simulink model "s9_3"  (R2024a)
settings: Solver=ode23  StartTime=0.0  StopTime=t_d  MaxStep=Tc  RelTol=1e-8  AbsTol=1e-8
model workspace: external: MAT-File C:\Users\tatwi\Documents\GitHub\robot_sim\Impedance_Control\test.mat (data not in the file)
values from neighbouring files (symbols this model uses):
  a = str2num(a_Field.Value)    [ImpedanceButton_Callback.m]    (also in i9_a_Backup.m = [1;1]; impedanceControl_ws.mat = [2 1]; param.m = [1;1]; test.mat = [1 1])
  F_v = K_r*diag([0.01 0.01])*K_r    [ImpedanceButton_Callback.m]    (also in i9_3.m; i9_a_Backup.m; impedanceControl_ws.mat = [100  0; 0  100]; test.mat = [100  0; 0  100])
  g = str2num(g_Field.Value)    [ImpedanceButton_Callback.m]    (also in i9_3.m = 9.81; i9_a_Backup.m = 9.81; impedanceControl_ws.mat = 9.81; test.mat = 9.81)
  iM_d = inv(M_d)    [ImpedanceButton_Callback.m]    (also in i9_3.m; i9_a_Backup.m; impedanceControl_ws.mat = [0.01  0; 0  0.01]; test.mat = [0.01  0; 0  0.01])
  K = R_c*[0 0;0 5e3]*R_c'    [ImpedanceButton_Callback.m]    (also in i9_3.m; i9_a_Backup.m; impedanceControl_ws.mat = [2500  -2500; -2500  2500]; test.mat = [2500  -2500; -2500  2500])
  K_d = Kd*diag([1 1])    [ImpedanceButton_Callback.m]    (also in i9_3.m = 1600*diag([1 1]); i9_a_Backup.m = 1600*diag([1 1]); impedanceControl_ws.mat = [1600  0; 0  1600]; test.mat = [1600  0; 0  1600])
  K_p = Kp*diag([1 1])    [ImpedanceButton_Callback.m]    (also in i9_3.m = 5000*diag([1 1]); i9_a_Backup.m = 5000*diag([1 1]); impedanceControl_ws.mat = [5000  0; 0  5000]; test.mat = [5000  0; 0  5000])
  o_r = [1;0]    [ImpedanceButton_Callback.m]    (also in i9_3.m; i9_a_Backup.m; impedanceControl_ws.mat = [1 0]; test.mat = [1 0])
  pi_l = pi_m    [ImpedanceButton_Callback.m]    (also in i9_3.m; i9_a_Backup.m; impedanceControl_ws.mat = [135 72.51 25 -2.5 0.01]; test.mat = [80 97.51 25 -2.5 0.01])
  pi_m = [135 72.51 25 -2.5 0.01]    [impedanceControl_ws.mat]    (also in test.mat = [80 97.51 25 -2.5 0.01])
  q_i = inv_k2u(a,p_i)    [ImpedanceButton_Callback.m]    (also in i9_3.m; i9_a_Backup.m; impedanceControl_ws.mat = [0.340969724421 -2.74996579108]; test.mat = [0.963425266026 -1.92685053205])
  Tc = str2num(tc_Field.Value)    [ImpedanceButton_Callback.m]    (also in i9_3.m = 0.001; i9_a_Backup.m = 0.001; impedanceControl_ws.mat = 0.001; test.mat = 0.001)
  Ts = Tc    [ImpedanceButton_Callback.m]    (also in i9_3.m = 0.001; i9_a_Backup.m = 0.001; impedanceControl_ws.mat = 0.001; test.mat = 0.001)
undefined symbols (not defined in the file or in its folder): iner, iner_l
settings Model: Creator=luigivillani  LastModifiedBy=tatwi
settings SolverCC: AutoScaleAbsTol=off  AlgebraicLoopSolver=TrustRegion
settings DataIOCC: SaveFormat=Array  SignalLoggingSaveFormat=ModelDataLogs  SaveOutput=off  SaveTime=off  ReturnWorkspaceOutputs=off
settings OptimizationCC: BlockReduction=off  BooleanDataType=off  ExpressionDepthLimit=2147483647  InitFltsAndDblsToZero=on  LifeSpan=inf
settings DebuggingCC: SaveWithParameterizedLinksMsg=none  UnderspecifiedInitializationDetection=Classic  MergeDetectMultiDrivingBlocksExec=none  SignalResolutionControl=TryResolveAllWithWarning  MultiTaskDSMMsg=warning  MultiTaskCondExecSysMsg=none  FcnCallInpInsideContextMsg=warning  UnconnectedInputMsg=warning  UnconnectedOutputMsg=warning  UnconnectedLineMsg=warning  StateNameClashWarn=warning  SFUnexpectedBacktrackingDiag=warning  SFNoUnconditionalDefaultTransitionDiag=warning  SFExecutionAtInitializationDiag=none  ArithmeticOperatorsInVariantConditions=warning
settings HardwareCC: ProdBitPerPointer=32  ProdBitPerSizeT=32  ProdBitPerPtrDiffT=32  ProdLargestAtomicFloat=None  ProdIntDivRoundTo=Undefined  ProdEndianess=Unspecified  ProdWordSize=32  ProdHWDeviceType=32-bit Generic  TargetUnknown=on
settings ModelReferenceCC: PropagateSignalLabelsOutOfModel=off
settings RTWCC: GPUComputeCapability=3.5
settings CodeAppCC: StateflowObjectComments=on
settings GRTTargetCC: TargetFcnLib=ansi_tfl_tmw.mat  TargetLangStandard=C89/C90 (ANSI)  CombineOutputUpdateFcns=off  GRTInterface=on
settings ConfigComp: CovMetricSettings=dw  CovSaveCumulativeToWorkspaceVar=on  CovSaveSingleToWorkspaceVar=on

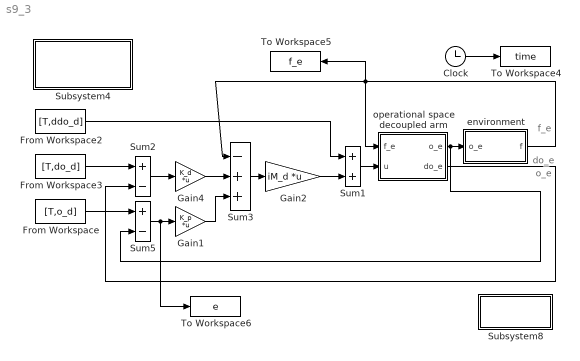
== system s9_3 ==
  note: o_e
  note: do_e
  note: f_e
  Clock : Clock
  From Workspace : FromWorkspace  VariableName=[T,o_d]  SampleTime=Tc  ZeroCross=off
  From Workspace2 : FromWorkspace  VariableName=[T,ddo_d]  SampleTime=Tc  ZeroCross=off
  From Workspace3 : FromWorkspace  VariableName=[T,do_d]  SampleTime=Tc  ZeroCross=off
  Gain1 : Gain  Gain=K_p  Multiplication=Matrix(K*u)  SampleTime=Tc
      mask Display: disp('K_p')
  Gain2 : Gain  Gain=iM_d  Multiplication=Matrix(K*u)  SampleTime=Tc
      mask Display: disp('inv(M_d)')
  Gain4 : Gain  Gain=K_d  Multiplication=Matrix(K*u)  SampleTime=Tc
      mask Display: disp('K_d')
  Subsystem4 : Subsystem
      settings: OpenFcn=clear all;i9_3;
      mask Display: disp('variables\ninitialization')
  Subsystem8 : Subsystem
      settings: OpenFcn=p9_3;
      mask Display: disp('plot')
  Sum1 : Sum  InputSameDT=on  SaturateOnIntegerOverflow=on  OutDataTypeStr=Inherit: Same as first input
  Sum2 : Sum  Inputs=+-  InputSameDT=on  SaturateOnIntegerOverflow=on  SampleTime=Tc  OutDataTypeStr=Inherit: Same as first input
  Sum3 : Sum  Inputs=-++  InputSameDT=on  SaturateOnIntegerOverflow=on  SampleTime=Tc  OutDataTypeStr=Inherit: Same as first input
  Sum5 : Sum  Inputs=+-  InputSameDT=on  SaturateOnIntegerOverflow=on  SampleTime=Tc  OutDataTypeStr=Inherit: Same as first input
  To Workspace4 : ToWorkspace  VariableName=time  SampleTime=Ts
      settings: MaxDataPoints=5001
  To Workspace5 : ToWorkspace  VariableName=f_e  SampleTime=Ts
      settings: MaxDataPoints=5001
  To Workspace6 : ToWorkspace  VariableName=e  SampleTime=Ts
      settings: MaxDataPoints=5001
  environment : Subsystem
      mask Display: disp('K(o_e-o_r)')
  operational space decoupled arm : Subsystem
      mask Display: disp('u = ddo_e')
  wires:
  Sum2/1 -> Gain4/1
  Sum5/1 -> Gain1/1, To Workspace6/1
  environment/1(f) -> operational space decoupled arm/1(f_e), Sum3/1, To Workspace5/1
  Clock/1 -> To Workspace4/1
  operational space decoupled arm/1(o_e) -> environment/1(o_e), Sum5/2
  operational space decoupled arm/2(do_e) -> Sum2/2
  From Workspace/1 -> Sum5/1
  From Workspace3/1 -> Sum2/1
  Gain4/1 -> Sum3/2
  Gain1/1 -> Sum3/3
  Sum3/1 -> Gain2/1
  Gain2/1 -> Sum1/2
  Sum1/1 -> operational space decoupled arm/2(u)
  From Workspace2/1 -> Sum1/1

== system s9_3/Subsystem4 ==
  note: start

== system s9_3/Subsystem8 ==
  note: start

== system s9_3/environment ==
  o_e : Inport
  Matrix gain. : StateSpace  A=[]  B=[]  C=[]  D=K  InitialCondition=0  mask(Matrix gain){K=K}
      mask prompts: K "Gain matrix:"
      mask help: Matrix Gain.
      mask Help: Multiplies input vector by entered matrix to produce output vector (y=Au).
      mask Display: disp('K')
  Sum1 : Sum  Inputs=+-  InputSameDT=on  SaturateOnIntegerOverflow=on  OutDataTypeStr=Inherit: Same as first input
  xo : Constant  Value=o_r
  f : Outport  InitialOutput=0
  wires:
  xo/1 -> Sum1/2
  Sum1/1 -> Matrix gain./1
  Matrix gain./1 -> f/1
  o_e/1 -> Sum1/1

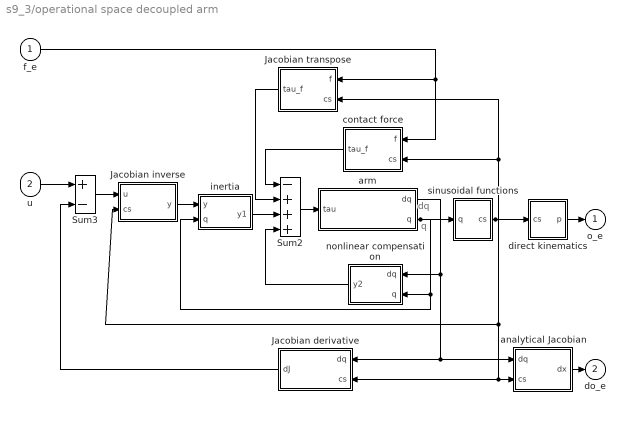
== system s9_3/operational space decoupled arm ==
  note: q
  note: dq
  f_e : Inport
  u : Inport  Port=2
  Jacobian derivative : Subsystem
      mask Display: disp('dJ_a(q,dq)')
  Jacobian inverse : Subsystem
      mask Display: disp('inv(J_a(q))')
  Jacobian transpose : Subsystem
      mask Display: disp('tr(J_a(q))')
  Sum2 : Sum  Inputs=-+++  InputSameDT=on  SaturateOnIntegerOverflow=on  OutDataTypeStr=Inherit: Same as first input
  Sum3 : Sum  Inputs=+-  InputSameDT=on  SaturateOnIntegerOverflow=on  OutDataTypeStr=Inherit: Same as first input
  analytical Jacobian : Subsystem
      mask Display: disp('J_a(q)')
  arm : Subsystem
      mask Display: disp('inv(B(q))(tau-tau'')')
  contact force : Subsystem
      mask Display: disp('tr(J_a(q))f')
  direct kinematics : Subsystem
      mask Display: disp('k(q)')
  inertia : Subsystem
      mask Display: disp('B(q)')
  nonlinear compensation : Subsystem
      mask Display: disp('n(q,dq)')
  sinusoidal functions : Subsystem
      mask Display: disp('cs(q)')
  o_e : Outport  InitialOutput=0
  do_e : Outport  Port=2  InitialOutput=0
  wires:
  Jacobian inverse/1(y) -> inertia/1(y)
  Sum2/1 -> arm/1(tau)
  arm/1(dq) -> analytical Jacobian/1(dq), Jacobian derivative/1(dq), nonlinear compensation/1(dq)
  direct kinematics/1(p) -> o_e/1
  analytical Jacobian/1(dx) -> do_e/1
  Sum3/1 -> Jacobian inverse/1(u)
  arm/2("q ") -> sinusoidal functions/1(q), nonlinear compensation/2(q), inertia/2(q)
  contact force/1(tau_f) -> Sum2/1
  sinusoidal functions/1(cs) -> direct kinematics/1(cs), contact force/2(cs), Jacobian transpose/2(cs), analytical Jacobian/2(cs), Jacobian derivative/2(cs), Jacobian inverse/2(cs)
  u/1 -> Sum3/1
  Jacobian derivative/1(dJ) -> Sum3/2
  nonlinear compensation/1(y2) -> Sum2/4
  inertia/1(y1) -> Sum2/3
  Jacobian transpose/1(tau_f) -> Sum2/2
  f_e/1 -> Jacobian transpose/1(f), contact force/1(f)

== system s9_3/operational space decoupled arm/Jacobian derivative ==
  dq : Inport
  cs : Inport  Port=2
  MATLAB Fcn : MATLABFcn  MATLABFcn=dJ_a  OutputDimensions=2  SampleTime=Tc
      mask Display: disp('dJ_a(q,dq)dq')
  Mux : Mux  Inputs=[2,4]
  dJ : Outport  InitialOutput=0
  wires:
  dq/1 -> Mux/1
  cs/1 -> Mux/2
  Mux/1 -> MATLAB Fcn/1
  MATLAB Fcn/1 -> dJ/1

== system s9_3/operational space decoupled arm/Jacobian inverse ==
  u : Inport
  cs : Inport  Port=2
  MATLAB Fcn : MATLABFcn  MATLABFcn=invJ_a  OutputDimensions=2  SampleTime=Tc
      mask Display: disp('inv(J_a(q))')
  Mux : Mux  Inputs=[2,4]
  y : Outport  InitialOutput=0
  wires:
  MATLAB Fcn/1 -> y/1
  Mux/1 -> MATLAB Fcn/1
  cs/1 -> Mux/2
  u/1 -> Mux/1

== system s9_3/operational space decoupled arm/Jacobian transpose ==
  f : Inport
  cs : Inport  Port=2
  MATLAB Fcn : MATLABFcn  MATLABFcn=trJ_a  OutputDimensions=2  SampleTime=Tc
      mask Display: disp('J''_a(q)f')
  Mux : Mux  Inputs=[2,4]
  tau_f : Outport  InitialOutput=0
  wires:
  MATLAB Fcn/1 -> tau_f/1
  Mux/1 -> MATLAB Fcn/1
  f/1 -> Mux/1
  cs/1 -> Mux/2

== system s9_3/operational space decoupled arm/analytical Jacobian ==
  dq : Inport
  cs : Inport  Port=2
  MATLAB Fcn : MATLABFcn  MATLABFcn=J_adq  OutputDimensions=2
      mask Display: disp('J_a(q)dq')
  Mux : Mux  Inputs=[2,4]
  dx : Outport  InitialOutput=0
  wires:
  dq/1 -> Mux/1
  Mux/1 -> MATLAB Fcn/1
  MATLAB Fcn/1 -> dx/1
  cs/1 -> Mux/2

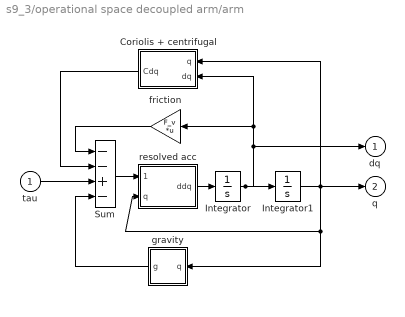
== system s9_3/operational space decoupled arm/arm ==
  tau : Inport
  Coriolis + centrifugal : Subsystem
      mask Display: disp('C(q,dq)dq')
  Integrator : Integrator  InitialCondition=[0 0]  ZeroCross=off
  Integrator1 : Integrator  InitialCondition=q_i  ZeroCross=off
  Sum : Sum  Inputs=--+-  InputSameDT=on  SaturateOnIntegerOverflow=on  OutDataTypeStr=Inherit: Same as first input
  friction : Gain  Gain=F_v  Multiplication=Matrix(K*u)  SaturateOnIntegerOverflow=on  OutDataTypeStr=Inherit: Same as input  ParamDataTypeStr=Inherit: Same as input
      mask Display: disp('F_v')
  gravity : Subsystem
      mask Display: disp('g(q)')
  resolved acc : Subsystem
      mask Display: disp('inv(B(q))')
  dq : Outport  InitialOutput=0
  "q " : Outport  Port=2  InitialOutput=0
  wires:
  Coriolis + centrifugal/1(Cdq) -> Sum/2
  tau/1 -> Sum/3
  Integrator1/1 -> Coriolis + centrifugal/1(q), resolved acc/2(q), gravity/1(q), "q "/1
  resolved acc/1(ddq) -> Integrator/1
  Integrator/1 -> Integrator1/1, dq/1, Coriolis + centrifugal/2(dq), friction/1
  Sum/1 -> resolved acc/1(tau-tau')
  friction/1 -> Sum/1
  gravity/1(g) -> Sum/4

== system s9_3/operational space decoupled arm/contact force ==
  f : Inport
  cs : Inport  Port=2
  MATLAB Fcn : MATLABFcn  MATLABFcn=trJ_a  OutputDimensions=2
      mask Display: disp('J''_a(q)f')
  Mux : Mux  Inputs=[2,4]
  tau_f : Outport  InitialOutput=0
  wires:
  f/1 -> Mux/1
  cs/1 -> Mux/2
  Mux/1 -> MATLAB Fcn/1
  MATLAB Fcn/1 -> tau_f/1

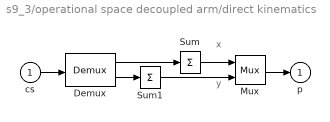
== system s9_3/operational space decoupled arm/direct kinematics ==
  note: x
  note: y
  cs : Inport
  Demux : Demux  Outputs=[2,2]
      settings: DisplayOption=none
  Mux : Mux  Inputs=2
  Sum : Sum  Inputs=+  InputSameDT=on  SaturateOnIntegerOverflow=on  OutDataTypeStr=Inherit: Same as first input
  Sum1 : Sum  Inputs=+  InputSameDT=on  SaturateOnIntegerOverflow=on  OutDataTypeStr=Inherit: Same as first input
  p : Outport  InitialOutput=0
  wires:
  Sum1/1 -> Mux/2
  Sum/1 -> Mux/1
  Demux/2 -> Sum1/1
  Demux/1 -> Sum/1
  cs/1 -> Demux/1
  Mux/1 -> p/1

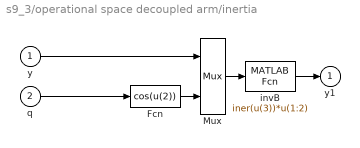
== system s9_3/operational space decoupled arm/inertia ==
  y : Inport
  q : Inport  Port=2
  Fcn : Fcn  Expr=cos(u(2))  SampleTime=Tc
  Mux : Mux  Inputs=[2,1]
  "invB " : MATLABFcn  MATLABFcn=iner(u(3))*u(1:2)  OutputDimensions=2  SampleTime=Tc
      mask Display: disp('B(q)y')
  y1 : Outport  InitialOutput=0
  wires:
  Fcn/1 -> Mux/2
  "invB "/1 -> y1/1
  Mux/1 -> "invB "/1
  q/1 -> Fcn/1
  y/1 -> Mux/1

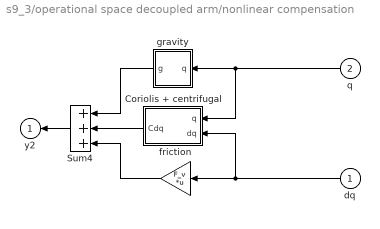
== system s9_3/operational space decoupled arm/nonlinear compensation ==
  dq : Inport
  q : Inport  Port=2
  Coriolis + centrifugal : Subsystem
      mask Display: disp('C(q,dq)dq')
  Sum4 : Sum  Inputs=+++  InputSameDT=on  SaturateOnIntegerOverflow=on  OutDataTypeStr=Inherit: Same as first input
  friction : Gain  Gain=F_v  Multiplication=Matrix(K*u)  SaturateOnIntegerOverflow=on  SampleTime=Tc  OutDataTypeStr=Inherit: Same as input  ParamDataTypeStr=Inherit: Same as input
      mask Display: disp('F_v')
  gravity : Subsystem
      mask Display: disp('g(q)')
  y2 : Outport  InitialOutput=0
  wires:
  gravity/1(g) -> Sum4/1
  Sum4/1 -> y2/1
  friction/1 -> Sum4/3
  q/1 -> gravity/1(q), Coriolis + centrifugal/1(q)
  dq/1 -> Coriolis + centrifugal/2(dq), friction/1
  Coriolis + centrifugal/1(Cdq) -> Sum4/2

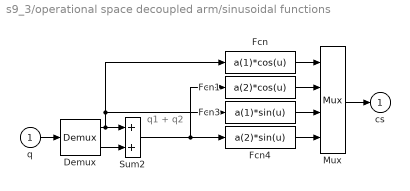
== system s9_3/operational space decoupled arm/sinusoidal functions ==
  note: q1 + q2
  q : Inport
  Demux : Demux  Outputs=2
      settings: DisplayOption=none
  Fcn : Fcn  Expr=a(1)*cos(u)
  Fcn1 : Fcn  Expr=a(2)*cos(u)
  Fcn3 : Fcn  Expr=a(1)*sin(u)
  Fcn4 : Fcn  Expr=a(2)*sin(u)
  Mux : Mux
  Sum2 : Sum  InputSameDT=on  SaturateOnIntegerOverflow=on  OutDataTypeStr=Inherit: Same as first input
  cs : Outport  InitialOutput=0
  wires:
  q/1 -> Demux/1
  Fcn4/1 -> Mux/4
  Fcn3/1 -> Mux/3
  Fcn1/1 -> Mux/2
  Sum2/1 -> Fcn1/1, Fcn4/1
  Demux/2 -> Sum2/2
  Demux/1 -> Fcn/1, Fcn3/1, Sum2/1
  Mux/1 -> cs/1
  Fcn/1 -> Mux/1

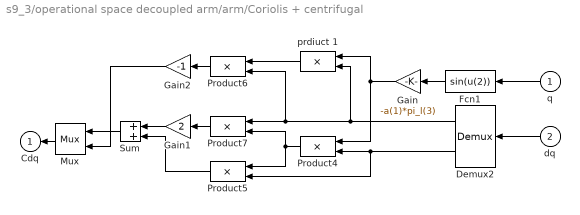
== system s9_3/operational space decoupled arm/arm/Coriolis + centrifugal ==
  q : Inport
  dq : Inport  Port=2
  Demux2 : Demux  Outputs=2
      settings: DisplayOption=none
  Fcn1 : Fcn  Expr=sin(u(2))
  Gain : Gain  Gain=-a(1)*pi_l(3)  SaturateOnIntegerOverflow=on  OutDataTypeStr=Inherit: Same as input  ParamDataTypeStr=Inherit: Same as input
      mask Display: disp('k_3')
  Gain1 : Gain  Gain=2  SaturateOnIntegerOverflow=on  OutDataTypeStr=Inherit: Same as input  ParamDataTypeStr=Inherit: Same as input
  Gain2 : Gain  Gain=-1  SaturateOnIntegerOverflow=on  OutDataTypeStr=Inherit: Same as input  ParamDataTypeStr=Inherit: Same as input
  Mux : Mux  Inputs=2
  Product{4..7} (4 alike) : Product  InputSameDT=on  RndMeth=Zero  SaturateOnIntegerOverflow=on  OutDataTypeStr=Inherit: Same as first input
  Sum : Sum  InputSameDT=on  SaturateOnIntegerOverflow=on  OutDataTypeStr=Inherit: Same as first input
  prdiuct 1 : Product  InputSameDT=on  RndMeth=Zero  SaturateOnIntegerOverflow=on  OutDataTypeStr=Inherit: Same as first input
  Cdq : Outport  InitialOutput=0
  wires:
  dq/1 -> Demux2/1
  Gain2/1 -> Mux/2
  Product6/1 -> Gain2/1
  Mux/1 -> Cdq/1
  Sum/1 -> Mux/1
  Product5/1 -> Sum/2
  Gain1/1 -> Sum/1
  Product7/1 -> Gain1/1
  Demux2/1 -> prdiuct 1/2, Product6/2, Product7/1
  Demux2/2 -> Product4/2, Product5/2
  prdiuct 1/1 -> Product6/1
  Gain/1 -> prdiuct 1/1, Product4/1
  Fcn1/1 -> Gain/1
  q/1 -> Fcn1/1
  Product4/1 -> Product5/1, Product7/2

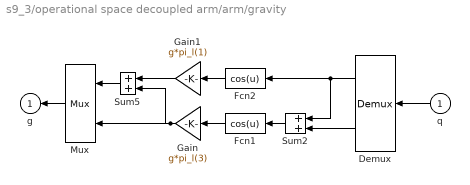
== system s9_3/operational space decoupled arm/arm/gravity ==
  q : Inport
  Demux : Demux  Outputs=2
      settings: DisplayOption=none
  Fcn1 : Fcn  Expr=cos(u)
  Fcn2 : Fcn  Expr=cos(u)
  Gain : Gain  Gain=g*pi_l(3)  SaturateOnIntegerOverflow=on  OutDataTypeStr=Inherit: Same as input  ParamDataTypeStr=Inherit: Same as input
      mask Display: disp('k_2')
  Gain1 : Gain  Gain=g*pi_l(1)  SaturateOnIntegerOverflow=on  OutDataTypeStr=Inherit: Same as input  ParamDataTypeStr=Inherit: Same as input
      mask Display: disp('k_1')
  Mux : Mux  Inputs=2
  Sum2 : Sum  InputSameDT=on  SaturateOnIntegerOverflow=on  OutDataTypeStr=Inherit: Same as first input
  Sum5 : Sum  InputSameDT=on  SaturateOnIntegerOverflow=on  OutDataTypeStr=Inherit: Same as first input
  g : Outport  InitialOutput=0
  wires:
  q/1 -> Demux/1
  Demux/2 -> Sum2/2
  Sum2/1 -> Fcn1/1
  Fcn1/1 -> Gain/1
  Fcn2/1 -> Gain1/1
  Demux/1 -> Fcn2/1, Sum2/1
  Gain1/1 -> Sum5/1
  Sum5/1 -> Mux/1
  Gain/1 -> Sum5/2, Mux/2
  Mux/1 -> g/1

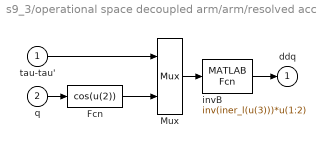
== system s9_3/operational space decoupled arm/arm/resolved acc ==
  tau-tau' : Inport
  q : Inport  Port=2
  Fcn : Fcn  Expr=cos(u(2))
  Mux : Mux  Inputs=[2,1]
  "invB " : MATLABFcn  MATLABFcn=inv(iner_l(u(3)))*u(1:2)  OutputDimensions=2
      mask Display: disp('inv(B(q))')
  ddq : Outport  InitialOutput=0
  wires:
  Fcn/1 -> Mux/2
  q/1 -> Fcn/1
  "invB "/1 -> ddq/1
  tau-tau'/1 -> Mux/1
  Mux/1 -> "invB "/1

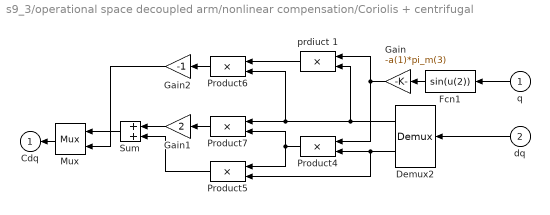
== system s9_3/operational space decoupled arm/nonlinear compensation/Coriolis + centrifugal ==
  q : Inport
  dq : Inport  Port=2
  Demux2 : Demux  Outputs=2
      settings: DisplayOption=none
  Fcn1 : Fcn  Expr=sin(u(2))  SampleTime=Tc
  Gain : Gain  Gain=-a(1)*pi_m(3)  SaturateOnIntegerOverflow=on  OutDataTypeStr=Inherit: Same as input  ParamDataTypeStr=Inherit: Same as input
      mask Display: disp('k_3')
  Gain1 : Gain  Gain=2  SaturateOnIntegerOverflow=on  OutDataTypeStr=Inherit: Same as input  ParamDataTypeStr=Inherit: Same as input
  Gain2 : Gain  Gain=-1  SaturateOnIntegerOverflow=on  OutDataTypeStr=Inherit: Same as input  ParamDataTypeStr=Inherit: Same as input
  Mux : Mux  Inputs=2
  Product{4..7} (4 alike) : Product  InputSameDT=on  RndMeth=Zero  SaturateOnIntegerOverflow=on  SampleTime=Tc  OutDataTypeStr=Inherit: Same as first input
  Sum : Sum  InputSameDT=on  SaturateOnIntegerOverflow=on  OutDataTypeStr=Inherit: Same as first input
  prdiuct 1 : Product  InputSameDT=on  RndMeth=Zero  SaturateOnIntegerOverflow=on  SampleTime=Tc  OutDataTypeStr=Inherit: Same as first input
  Cdq : Outport  InitialOutput=0
  wires:
  Product4/1 -> Product5/1, Product7/2
  Demux2/1 -> prdiuct 1/2, Product6/2, Product7/1
  Fcn1/1 -> Gain/1
  Gain/1 -> prdiuct 1/1, Product4/1
  prdiuct 1/1 -> Product6/1
  Product7/1 -> Gain1/1
  Gain1/1 -> Sum/1
  Product5/1 -> Sum/2
  Sum/1 -> Mux/1
  Mux/1 -> Cdq/1
  Product6/1 -> Gain2/1
  Gain2/1 -> Mux/2
  q/1 -> Fcn1/1
  dq/1 -> Demux2/1
  Demux2/2 -> Product4/2, Product5/2

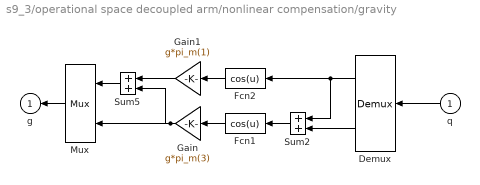
== system s9_3/operational space decoupled arm/nonlinear compensation/gravity ==
  q : Inport
  Demux : Demux  Outputs=2
      settings: DisplayOption=none
  Fcn1 : Fcn  Expr=cos(u)  SampleTime=Tc
  Fcn2 : Fcn  Expr=cos(u)  SampleTime=Tc
  Gain : Gain  Gain=g*pi_m(3)  SaturateOnIntegerOverflow=on  OutDataTypeStr=Inherit: Same as input  ParamDataTypeStr=Inherit: Same as input
      mask Display: disp('k_2')
  Gain1 : Gain  Gain=g*pi_m(1)  SaturateOnIntegerOverflow=on  OutDataTypeStr=Inherit: Same as input  ParamDataTypeStr=Inherit: Same as input
      mask Display: disp('k_1')
  Mux : Mux  Inputs=2
  Sum2 : Sum  InputSameDT=on  SaturateOnIntegerOverflow=on  SampleTime=Tc  OutDataTypeStr=Inherit: Same as first input
  Sum5 : Sum  InputSameDT=on  SaturateOnIntegerOverflow=on  OutDataTypeStr=Inherit: Same as first input
  g : Outport  InitialOutput=0
  wires:
  q/1 -> Demux/1
  Demux/2 -> Sum2/2
  Sum2/1 -> Fcn1/1
  Fcn1/1 -> Gain/1
  Fcn2/1 -> Gain1/1
  Demux/1 -> Fcn2/1, Sum2/1
  Gain1/1 -> Sum5/1
  Sum5/1 -> Mux/1
  Gain/1 -> Mux/2, Sum5/2
  Mux/1 -> g/1
